simulink subsystem "f_meas"  (R2022a)
settings: Solver=VariableStepAuto  StartTime=0.0  StopTime=10.0  RelTol=1e-3
values from neighbouring files (symbols this model uses):
  a0 = 1    [sim3run_390.m]
  a1 = -2*2*tau/(2*tau+3)    (= -1.96531791908)    [sim3run_390.m]
  a2 = 2*tau*(2*tau+1)/((2*tau+3)*(2*tau+3+1))    (= 0.965716563683)    [sim3run_390.m]
  ControlSampleTime = 1/8000    (= 0.000125)    [sim3run_390.m]
  Rco_gain = tau*ControlSampleTime    (= 0.010625)    [sim3run_390.m]
  Rco_lim = 4    [sim3run_390.m]
  Rco_Tint = 0.001    [sim3run_390.m]
undefined symbols (not defined in the file or in its folder): DiscIntNeverNeededParam, General, VSM
libraries: ee_lib x6, FriedrichLibrary x6, nesl_utility x3, simulink x2, spsPower3phInstantaneousLib x1
settings Model: Creator=uk062294  LastModifiedBy=uk062294
settings ModelReferenceCC: EnableRefExpFcnMdlSchedulingChecks=off
settings RTWCC: Description=Generic Real-Time Target

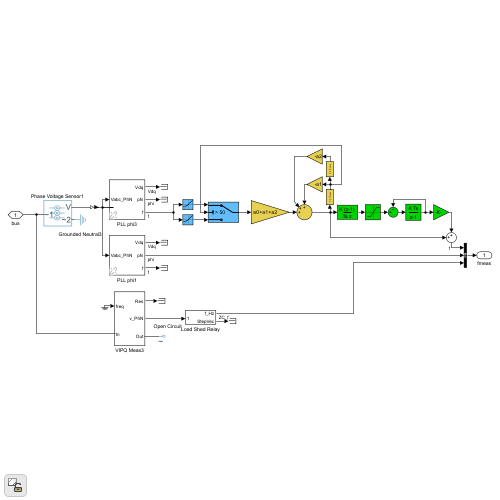
[thumbnail: Simulink's stored preview of the top-level diagram]
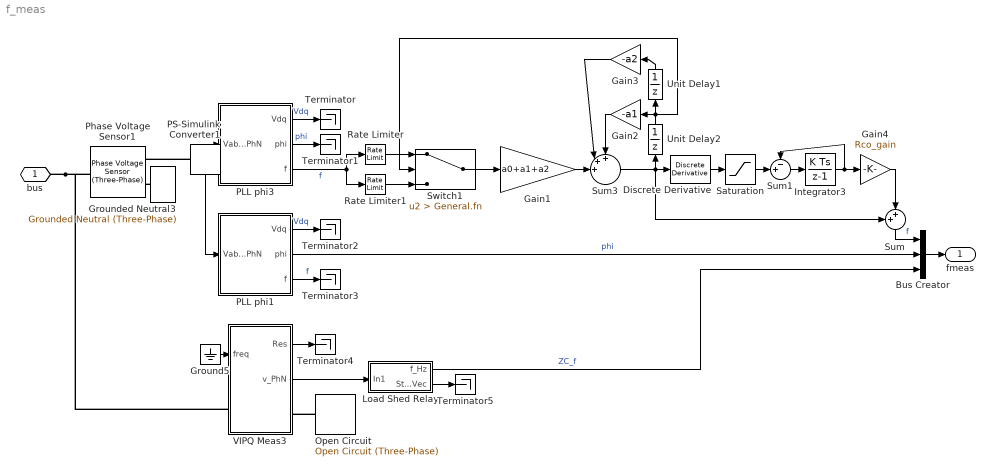
== system f_meas ==
  Bus Creator : BusCreator  Inputs=3
  Discrete Derivative : simulink/Discrete/Discrete Derivative  gainval=1.0  ICPrevScaledInput=0.0  OutMin=[]  OutMax=[]  OutDataType=fixdt(1, 16)  OutScaling=2^-10  DoSatur=off
  Gain1 : Gain  Gain=a0+a1+a2
  Gain2 : Gain  Gain=-a1
  Gain3 : Gain  Gain=-a2
  Gain4 : Gain  Gain=Rco_gain
  Ground5 : Ground
  Grounded Neutral3 : ee_lib/Connectors & References/Grounded Neutral (Three-Phase)
  Integrator3 : DiscreteIntegrator  gainval=1/Rco_Tint  InitialCondition=General.fn  SampleTime=ControlSampleTime  ICPrevOutput=DiscIntNeverNeededParam  ICPrevScaledInput=DiscIntNeverNeededParam
  Load Shed Relay : Subsystem
  Open Circuit : ee_lib/Connectors & References/Open Circuit (Three-Phase)
      settings: InternalSimscapePortConfiguration="{\"Bottom\":[],\"Left\":[{\"id\":\"N\",\"label\":\"~\",\"type\":\"foundation.electrical.three_phase\"}],\"Right\":[],\"Top\":[]}"
  PLL phi1 : Subsystem  AncestorBlock=FriedrichLibrary/Discrete Stuff/Symmetrical PLL  mask{Kp_PLL=VSM.PLLa.kp, Ki_PLL=VSM.PLLa.ki, Kd_PLL=0, Ts=ControlSampleTime}
      mask prompts: Kp_PLL "Proportional Gain PLL"; Ki_PLL "Integral Gain PLL"; Kd_PLL "Differential Gain PLL"; Ts "SampleTime"
      mask DialogControl DescGroupVar Prompt: SRF PLL
      mask DialogControl DescTextVar Prompt: Discrete implementation of a synchronous reference phase locked loop.
  PLL phi3 : Subsystem  AncestorBlock=FriedrichLibrary/Discrete Stuff/Symmetrical PLL  mask{Kp_PLL=VSM.PLLf.kp, Ki_PLL=VSM.PLLf.ki, Kd_PLL=0, Ts=ControlSampleTime}
      mask prompts: Kp_PLL "Proportional Gain PLL"; Ki_PLL "Integral Gain PLL"; Kd_PLL "Differential Gain PLL"; Ts "SampleTime"
      mask DialogControl DescGroupVar Prompt: SRF PLL
      mask DialogControl DescTextVar Prompt: Discrete implementation of a synchronous reference phase locked loop.
  PS-Simulink Converter1 : nesl_utility/PS-Simulink Converter  PhysicalDomain=network_engine_domain  SubClassName=ps_output  LeftPortType=input  RightPortType=output  PseudoPeriodic=off  Frequencies=[]  VectorFormat=1-D array  Unit=1  AffineConversion=off
  Phase Voltage Sensor1 : ee_lib/Sensors & Transducers/Phase Voltage Sensor (Three-Phase)
  Rate Limiter : RateLimiter  RisingSlewLimit=10  FallingSlewLimit=-1000  SampleTimeMode=inherited  InitialCondition=50
  Rate Limiter1 : RateLimiter  RisingSlewLimit=1000  FallingSlewLimit=-10  SampleTimeMode=inherited  InitialCondition=50
  Saturation : Saturate  UpperLimit=Rco_lim  LowerLimit=-Rco_lim
  Sum : Sum  Inputs=++|
  Sum1 : Sum  Inputs=-+|
  Sum3 : Sum  Inputs=+++||
  Switch1 : Switch  Criteria=u2 > Threshold  Threshold=General.fn  SaturateOnIntegerOverflow=off  InputSameDT=off
  Terminator{,1..5} (6 alike) : Terminator
  Unit Delay1 : UnitDelay  InitialCondition=General.fn  SampleTime=ControlSampleTime  HasFrameUpgradeWarning=on
  Unit Delay2 : UnitDelay  InitialCondition=General.fn  SampleTime=ControlSampleTime  HasFrameUpgradeWarning=on
  VIPQ Meas3 : Subsystem
  bus : PMIOPort  Side=Left
  fmeas : Outport  VectorParamsAs1DForOutWhenUnconnected=off
  wires:
  Ground5/1 -> VIPQ Meas3/1(freq)
  PLL phi3/1(Vdq) -> Terminator/1  "Vdq"
  VIPQ Meas3/2(v_PhN) -> Load Shed Relay/1(In1)
  Load Shed Relay/2(StepVec) -> Terminator5/1
  PS-Simulink Converter1/1 -> PLL phi1/1(Vabc_PhN), PLL phi3/1(Vabc_PhN)
  PLL phi1/3(f) -> Terminator3/1  "f"
  VIPQ Meas3/1(Res) -> Terminator4/1
  PLL phi1/1(Vdq) -> Terminator2/1  "Vdq"
  PLL phi3/2(phi) -> Terminator1/1  "phi"
  Gain2/1 -> Sum3/1
  Gain3/1 -> Sum3/2
  Unit Delay2/1 -> Gain2/1, Unit Delay1/1, Switch1/2
  Sum3/1 -> Unit Delay2/1, Sum/1, Discrete Derivative/1
  PLL phi1/2(phi) -> Bus Creator/2  "phi"
  Bus Creator/1 -> fmeas/1
  Unit Delay1/1 -> Gain3/1
  Gain1/1 -> Sum3/3
  Sum1/1 -> Integrator3/1
  Integrator3/1 -> Sum1/1, Gain4/1
  Sum/1 -> Bus Creator/1  "f"
  Discrete Derivative/1 -> Saturation/1
  Switch1/1 -> Gain1/1
  Gain4/1 -> Sum/2
  Saturation/1 -> Sum1/2
  PLL phi3/3(f) -> Rate Limiter/1, Rate Limiter1/1  "f"
  Load Shed Relay/1(f_Hz) -> Bus Creator/3  "ZC_f"
  Rate Limiter/1 -> Switch1/1
  Rate Limiter1/1 -> Switch1/3
  connections:
  bus/RConn1 -- Phase Voltage Sensor1/LConn1 -- VIPQ Meas3/LConn1
  Grounded Neutral3/LConn1 -- Phase Voltage Sensor1/RConn2
  PS-Simulink Converter1/LConn1 -- Phase Voltage Sensor1/RConn1
  Open Circuit/LConn1 -- VIPQ Meas3/RConn1

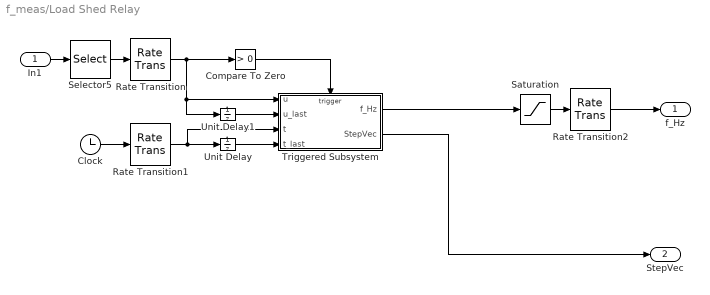
== system f_meas/Load Shed Relay ==
  In1 : Inport
  Clock : Clock
  Compare To Zero : simulink/Logic and Bit Operations/Compare To Zero  relop=>  OutDataTypeStr=boolean
  Rate Transition : RateTransition  OutPortSampleTime=ControlSampleTime
  Rate Transition1 : RateTransition  OutPortSampleTime=ControlSampleTime
  Rate Transition2 : RateTransition  OutPortSampleTime=ControlSampleTime
  Saturation : Saturate  UpperLimit=60  LowerLimit=40
  Selector5 : Selector  InputPortWidth=3  IndexOptions=Index vector (dialog)  Indices=1  OutputSizes=1
  Triggered Subsystem : Subsystem  TreatAsAtomicUnit=on
  Unit Delay : UnitDelay  SampleTime=-1  HasFrameUpgradeWarning=on
  Unit Delay1 : UnitDelay  SampleTime=-1  HasFrameUpgradeWarning=on
  f_Hz : Outport  VectorParamsAs1DForOutWhenUnconnected=off
  StepVec : Outport  Port=2  VectorParamsAs1DForOutWhenUnconnected=off
  wires:
  Triggered Subsystem/2(StepVec) -> StepVec/1
  Unit Delay/1 -> Triggered Subsystem/4(t_last)
  Rate Transition2/1 -> f_Hz/1
  Rate Transition/1 -> Compare To Zero/1, Unit Delay1/1, Triggered Subsystem/1(u)
  Saturation/1 -> Rate Transition2/1
  Selector5/1 -> Rate Transition/1
  Unit Delay1/1 -> Triggered Subsystem/2(u_last)
  Triggered Subsystem/1(f_Hz) -> Saturation/1
  In1/1 -> Selector5/1
  Compare To Zero/1 -> Triggered Subsystem/Trigger
  Clock/1 -> Rate Transition1/1
  Rate Transition1/1 -> Unit Delay/1, Triggered Subsystem/3(t)

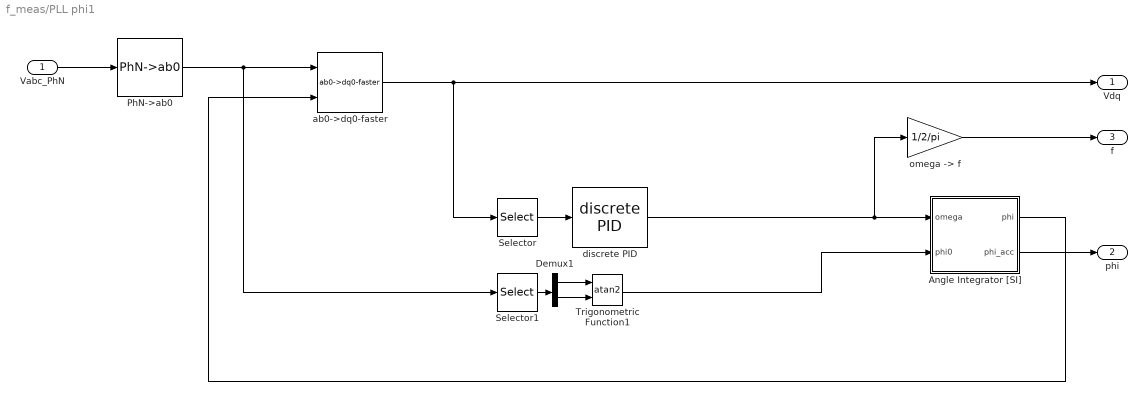
== system f_meas/PLL phi1 ==
  Vabc_PhN : Inport
  Angle Integrator [SI] : Subsystem  AncestorBlock=FriedrichLibrary/Discrete Stuff/Angle Integrator [SI]  mask{Ts=Ts}
      mask prompts: Ts "SampleTime"
      mask DialogControl DescGroupVar Prompt: Angle Integrator [SI]
      mask DialogControl DescTextVar Prompt: Discrete Integrator for omega, resetting every 2*pi.
  Demux1 : Demux  Outputs=2
  PhN->ab0 : FriedrichLibrary/Transformations/PhN->ab0  SystemSampleTime=-1  VariantActivationTime=update diagram  Latency=0  AutoFrameSizeCalculation=off
  Selector : Selector  InputPortWidth=3  IndexOptions=Index vector (dialog)  Indices=2  OutputSizes=1
  Selector1 : Selector  InputPortWidth=3  IndexOptions=Index vector (dialog)  Indices=[2 1]  OutputSizes=1
  Trigonometric Function1 : Trigonometry  Operator=atan2
  ab0->dq0-faster : FriedrichLibrary/Transformations/ab0->dq0-faster  SystemSampleTime=-1  VariantActivationTime=update diagram  Latency=0  AutoFrameSizeCalculation=off
  discrete PID : FriedrichLibrary/Discrete Stuff/discrete PID  Kp=Kp_PLL  Ki=Ki_PLL  Kd=Kd_PLL  Ts=Ts  x_init=2*pi*50
  "omega -> f" : Gain  Gain=1/2/pi
  Vdq : Outport  VectorParamsAs1DForOutWhenUnconnected=off
  phi : Outport  Port=2  VectorParamsAs1DForOutWhenUnconnected=off
  f : Outport  Port=3  VectorParamsAs1DForOutWhenUnconnected=off
  wires:
  Angle Integrator [SI]/2(phi_acc) -> phi/1
  Trigonometric Function1/1 -> Angle Integrator [SI]/2(phi0)
  Demux1/2 -> Trigonometric Function1/2
  Demux1/1 -> Trigonometric Function1/1
  Selector1/1 -> Demux1/1
  PhN->ab0/1 -> ab0->dq0-faster/1, Selector1/1
  Vabc_PhN/1 -> PhN->ab0/1
  "omega -> f"/1 -> f/1
  Angle Integrator [SI]/1(phi) -> ab0->dq0-faster/2
  discrete PID/1 -> "omega -> f"/1, Angle Integrator [SI]/1(omega)
  Selector/1 -> discrete PID/1
  ab0->dq0-faster/1 -> Selector/1, Vdq/1

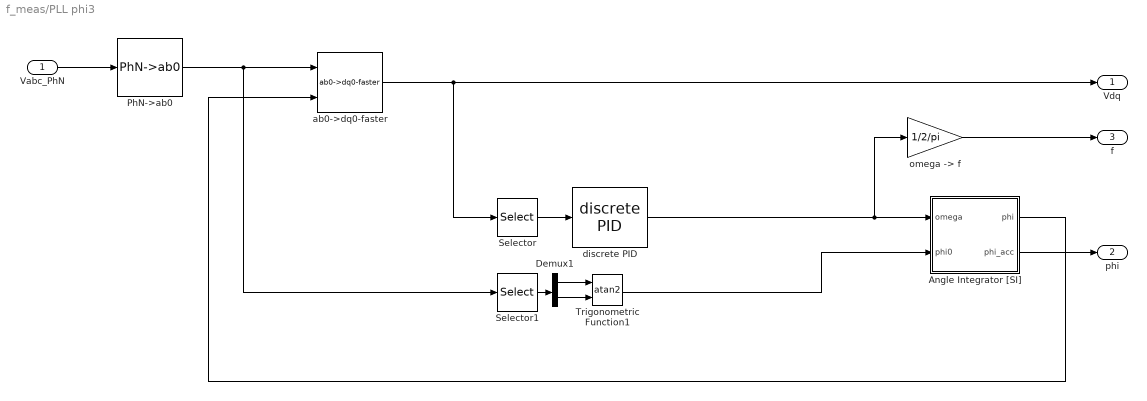
== system f_meas/PLL phi3 ==
  Vabc_PhN : Inport
  Angle Integrator [SI] : Subsystem  AncestorBlock=FriedrichLibrary/Discrete Stuff/Angle Integrator [SI]  mask{Ts=Ts}
      mask prompts: Ts "SampleTime"
      mask DialogControl DescGroupVar Prompt: Angle Integrator [SI]
      mask DialogControl DescTextVar Prompt: Discrete Integrator for omega, resetting every 2*pi.
  Demux1 : Demux  Outputs=2
  PhN->ab0 : FriedrichLibrary/Transformations/PhN->ab0  SystemSampleTime=-1  VariantActivationTime=update diagram  Latency=0  AutoFrameSizeCalculation=off
  Selector : Selector  InputPortWidth=3  IndexOptions=Index vector (dialog)  Indices=2  OutputSizes=1
  Selector1 : Selector  InputPortWidth=3  IndexOptions=Index vector (dialog)  Indices=[2 1]  OutputSizes=1
  Trigonometric Function1 : Trigonometry  Operator=atan2
  ab0->dq0-faster : FriedrichLibrary/Transformations/ab0->dq0-faster  SystemSampleTime=-1  VariantActivationTime=update diagram  Latency=0  AutoFrameSizeCalculation=off
  discrete PID : FriedrichLibrary/Discrete Stuff/discrete PID  Kp=Kp_PLL  Ki=Ki_PLL  Kd=Kd_PLL  Ts=Ts  x_init=2*pi*50
  "omega -> f" : Gain  Gain=1/2/pi
  Vdq : Outport  VectorParamsAs1DForOutWhenUnconnected=off
  phi : Outport  Port=2  VectorParamsAs1DForOutWhenUnconnected=off
  f : Outport  Port=3  VectorParamsAs1DForOutWhenUnconnected=off
  wires:
  Angle Integrator [SI]/2(phi_acc) -> phi/1
  Trigonometric Function1/1 -> Angle Integrator [SI]/2(phi0)
  Demux1/2 -> Trigonometric Function1/2
  Demux1/1 -> Trigonometric Function1/1
  Selector1/1 -> Demux1/1
  PhN->ab0/1 -> ab0->dq0-faster/1, Selector1/1
  Vabc_PhN/1 -> PhN->ab0/1
  "omega -> f"/1 -> f/1
  Angle Integrator [SI]/1(phi) -> ab0->dq0-faster/2
  discrete PID/1 -> "omega -> f"/1, Angle Integrator [SI]/1(omega)
  Selector/1 -> discrete PID/1
  ab0->dq0-faster/1 -> Selector/1, Vdq/1

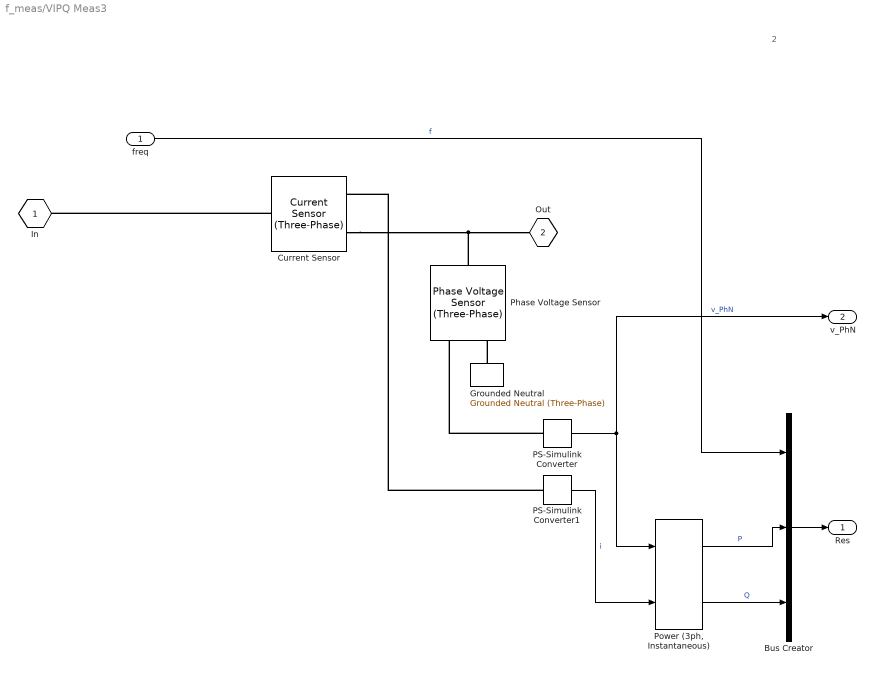
== system f_meas/VIPQ Meas3 ==
  note: 2
  freq : Inport
  Bus Creator : BusCreator  Inputs=3
  Current Sensor : ee_lib/Sensors & Transducers/Current Sensor (Three-Phase)
  Grounded Neutral : ee_lib/Connectors & References/Grounded Neutral (Three-Phase)
  PS-Simulink Converter : nesl_utility/PS-Simulink Converter  PhysicalDomain=network_engine_domain  SubClassName=ps_output  LeftPortType=input  RightPortType=output  PseudoPeriodic=off  Frequencies=[]  VectorFormat=1-D array  Unit=1  AffineConversion=off
  PS-Simulink Converter1 : nesl_utility/PS-Simulink Converter  PhysicalDomain=network_engine_domain  SubClassName=ps_output  LeftPortType=input  RightPortType=output  PseudoPeriodic=off  Frequencies=[]  VectorFormat=1-D array  Unit=1  AffineConversion=off
  Phase Voltage Sensor : ee_lib/Sensors & Transducers/Phase Voltage Sensor (Three-Phase)
  "Power (3ph, Instantaneous)" : spsPower3phInstantaneousLib/Power (3ph, Instantaneous)
  In : PMIOPort  Side=Left
  Out : PMIOPort  Port=2  Side=Right
  Res : Outport  VectorParamsAs1DForOutWhenUnconnected=off
  v_PhN : Outport  Port=2  VectorParamsAs1DForOutWhenUnconnected=off
  wires:
  freq/1 -> Bus Creator/1  "f"
  PS-Simulink Converter/1 -> v_PhN/1, "Power (3ph, Instantaneous)"/1  "v_PhN"
  PS-Simulink Converter1/1 -> "Power (3ph, Instantaneous)"/2  "i"
  "Power (3ph, Instantaneous)"/1 -> Bus Creator/2  "P"
  "Power (3ph, Instantaneous)"/2 -> Bus Creator/3  "Q"
  Bus Creator/1 -> Res/1
  connections:
  PS-Simulink Converter/LConn1 -- Phase Voltage Sensor/RConn1
  PS-Simulink Converter1/LConn1 -- Current Sensor/RConn1
  Grounded Neutral/LConn1 -- Phase Voltage Sensor/RConn2
  Phase Voltage Sensor/LConn1 -- Current Sensor/RConn2 -- Out/RConn1
  Current Sensor/LConn1 -- In/RConn1

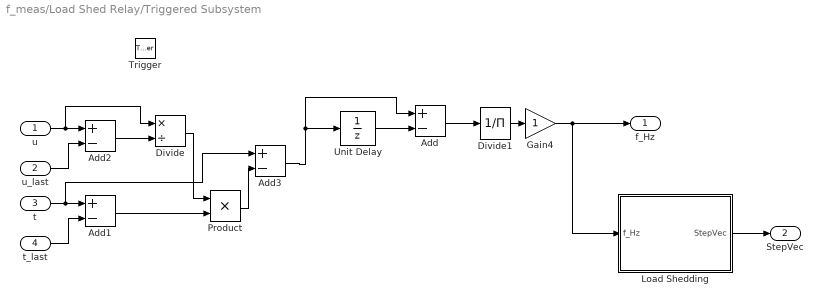
== system f_meas/Load Shed Relay/Triggered Subsystem ==
  u : Inport
  u_last : Inport  Port=2
  t : Inport  Port=3
  t_last : Inport  Port=4
  Trigger : TriggerPort  VariantControl=(inherit)
  Add{,1..3} (4 alike) : Sum  Inputs=+-
  Divide : Product  Inputs=*/
  Divide1 : Product  Inputs=/
  Gain4 : Gain
  "Load Shedding " : Subsystem  mask{f_shed_vec=[49 48.66 48.33 48]}
      mask prompts: f_shed_vec "Frequency level vector [Hz]"
      mask init:
      | ones_shed = ones(size(f_shed_vec));
  Product : Product
  Unit Delay : UnitDelay  SampleTime=-1  HasFrameUpgradeWarning=on
  f_Hz : Outport  VectorParamsAs1DForOutWhenUnconnected=off
  StepVec : Outport  Port=2  VectorParamsAs1DForOutWhenUnconnected=off
  wires:
  "Load Shedding "/1(StepVec) -> StepVec/1
  Gain4/1 -> f_Hz/1, "Load Shedding "/1(f_Hz)
  Divide1/1 -> Gain4/1
  Product/1 -> Add3/2
  Add1/1 -> Product/2
  Divide/1 -> Product/1
  Add2/1 -> Divide/2
  t_last/1 -> Add1/2
  t/1 -> Add1/1, Add3/1
  u_last/1 -> Add2/2
  u/1 -> Add2/1, Divide/1
  Add/1 -> Divide1/1
  Unit Delay/1 -> Add/2
  Add3/1 -> Unit Delay/1, Add/1

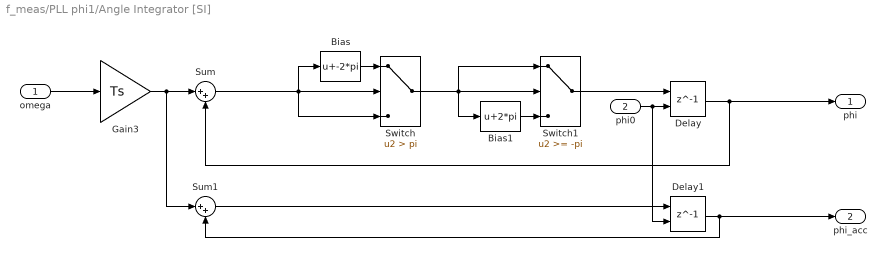
== system f_meas/PLL phi1/Angle Integrator [SI] ==
  omega : Inport
  phi0 : Inport  Port=2
  Bias : Bias  Bias=-2*pi  SaturateOnIntegerOverflow=off
  Bias1 : Bias  Bias=2*pi  SaturateOnIntegerOverflow=off
  Delay : Delay  DelayLength=1  InitialConditionSource=Input port  SampleTime=Ts
      settings: InputPortMap=u0,p4
  Delay1 : Delay  DelayLength=1  InitialConditionSource=Input port  SampleTime=Ts
      settings: InputPortMap=u0,p4
  Gain3 : Gain  Gain=Ts
  Sum : Sum  Inputs=|++
  Sum1 : Sum  Inputs=|++
  Switch : Switch  Criteria=u2 > Threshold  Threshold=pi  SaturateOnIntegerOverflow=off  InputSameDT=off
  Switch1 : Switch  Threshold=-pi  SaturateOnIntegerOverflow=off  InputSameDT=off
  phi : Outport  VectorParamsAs1DForOutWhenUnconnected=off
  phi_acc : Outport  Port=2  VectorParamsAs1DForOutWhenUnconnected=off
  wires:
  Sum1/1 -> Delay1/1
  Gain3/1 -> Sum/1, Sum1/1
  phi0/1 -> Delay/2, Delay1/2
  Delay1/1 -> Sum1/2, phi_acc/1
  omega/1 -> Gain3/1
  Bias/1 -> Switch/1
  Sum/1 -> Switch/3, Switch/2, Bias/1
  Delay/1 -> Sum/2, phi/1
  Switch/1 -> Switch1/1, Bias1/1, Switch1/2
  Bias1/1 -> Switch1/3
  Switch1/1 -> Delay/1

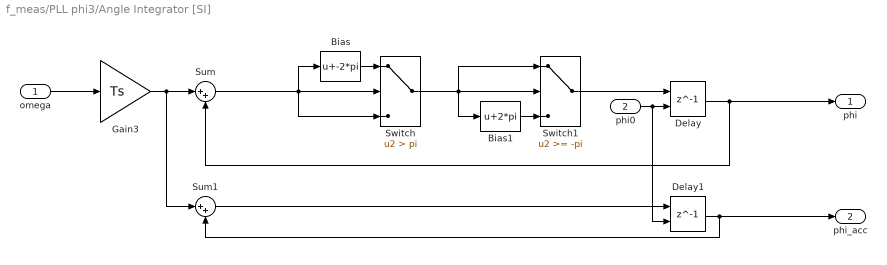
== system f_meas/PLL phi3/Angle Integrator [SI] ==
  omega : Inport
  phi0 : Inport  Port=2
  Bias : Bias  Bias=-2*pi  SaturateOnIntegerOverflow=off
  Bias1 : Bias  Bias=2*pi  SaturateOnIntegerOverflow=off
  Delay : Delay  DelayLength=1  InitialConditionSource=Input port  SampleTime=Ts
      settings: InputPortMap=u0,p4
  Delay1 : Delay  DelayLength=1  InitialConditionSource=Input port  SampleTime=Ts
      settings: InputPortMap=u0,p4
  Gain3 : Gain  Gain=Ts
  Sum : Sum  Inputs=|++
  Sum1 : Sum  Inputs=|++
  Switch : Switch  Criteria=u2 > Threshold  Threshold=pi  SaturateOnIntegerOverflow=off  InputSameDT=off
  Switch1 : Switch  Threshold=-pi  SaturateOnIntegerOverflow=off  InputSameDT=off
  phi : Outport  VectorParamsAs1DForOutWhenUnconnected=off
  phi_acc : Outport  Port=2  VectorParamsAs1DForOutWhenUnconnected=off
  wires:
  Sum1/1 -> Delay1/1
  Gain3/1 -> Sum/1, Sum1/1
  phi0/1 -> Delay/2, Delay1/2
  Delay1/1 -> Sum1/2, phi_acc/1
  omega/1 -> Gain3/1
  Bias/1 -> Switch/1
  Sum/1 -> Switch/3, Switch/2, Bias/1
  Delay/1 -> Sum/2, phi/1
  Switch/1 -> Switch1/1, Bias1/1, Switch1/2
  Bias1/1 -> Switch1/3
  Switch1/1 -> Delay/1

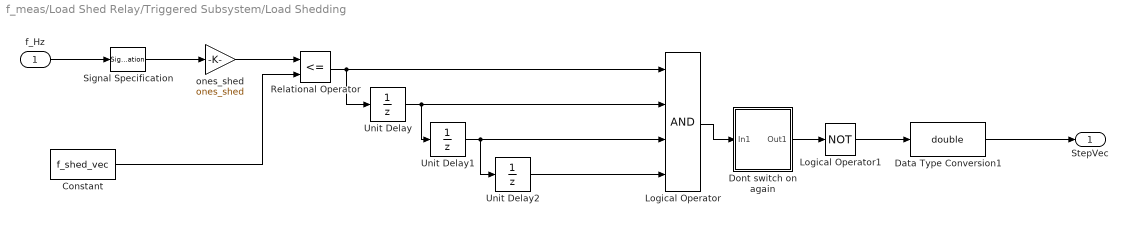
== system f_meas/Load Shed Relay/Triggered Subsystem/Load Shedding  ==
  f_Hz : Inport
  Constant : Constant  Value=f_shed_vec
  Data Type Conversion1 : DataTypeConversion  OutDataTypeStr=double  SaturateOnIntegerOverflow=off  RndMeth=Floor
  Dont switch on again : Subsystem
  Logical Operator : Logic  Inputs=4  AllPortsSameDT=off  OutDataTypeStr=boolean
  Logical Operator1 : Logic  Operator=NOT  Inputs=1  AllPortsSameDT=off  OutDataTypeStr=boolean
  Relational Operator : RelationalOperator  Operator=<=  OutDataTypeStr=boolean  InputSameDT=off
  Signal Specification : SignalSpecification  Dimensions=[1]
  Unit Delay : UnitDelay  SampleTime=-1  HasFrameUpgradeWarning=on
  Unit Delay1 : UnitDelay  SampleTime=-1  HasFrameUpgradeWarning=on
  Unit Delay2 : UnitDelay  SampleTime=-1  HasFrameUpgradeWarning=on
  ones_shed : Gain  Gain=ones_shed
  StepVec : Outport  VectorParamsAs1DForOutWhenUnconnected=off
  wires:
  Logical Operator1/1 -> Data Type Conversion1/1
  Logical Operator/1 -> Dont switch on again/1(In1)
  Unit Delay2/1 -> Logical Operator/4
  Unit Delay1/1 -> Logical Operator/3, Unit Delay2/1
  Unit Delay/1 -> Logical Operator/2, Unit Delay1/1
  Dont switch on again/1(Out1) -> Logical Operator1/1
  Data Type Conversion1/1 -> StepVec/1
  Relational Operator/1 -> Unit Delay/1, Logical Operator/1
  Signal Specification/1 -> ones_shed/1
  ones_shed/1 -> Relational Operator/1
  f_Hz/1 -> Signal Specification/1
  Constant/1 -> Relational Operator/2

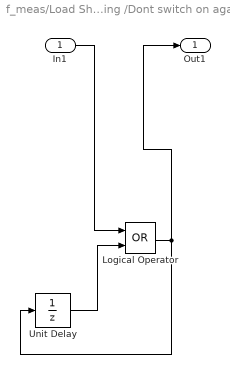
== system f_meas/Load Shed Relay/Triggered Subsystem/Load Shedding /Dont switch on again ==
  In1 : Inport
  Logical Operator : Logic  Operator=OR  AllPortsSameDT=off  OutDataTypeStr=boolean
  Unit Delay : UnitDelay  SampleTime=-1  HasFrameUpgradeWarning=on
  Out1 : Outport  VectorParamsAs1DForOutWhenUnconnected=off
  wires:
  Unit Delay/1 -> Logical Operator/2
  Logical Operator/1 -> Out1/1, Unit Delay/1
  In1/1 -> Logical Operator/1
